simulink model "step_response_firstorder_rl_rc"  (R2021a)
settings: Solver=VariableStepAuto  StartTime=0.0  StopTime=0.05  RelTol=1e-3
libraries: spsSeriesRLCBranchLib x12, spsControlledVoltageSourceLib x6, spsCurrentMeasurementLib x6, spsVoltageMeasurementLib x6, spspowerguiLib x1
settings Model: Creator=LENOVO  LastModifiedBy=LENOVO

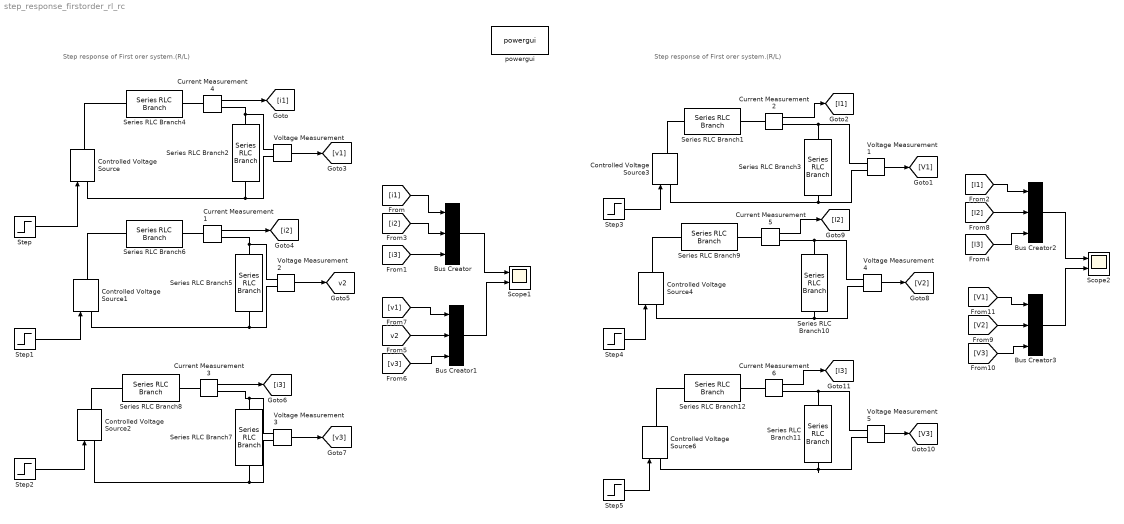
== system step_response_firstorder_rl_rc ==
  note: Step response of First orer system.(R/L)
  note: Step response of First orer system.(R/L)
  Bus Creator{,1..3} (4 alike) : BusCreator  Inputs=3
  Controlled Voltage Source{,1..4,6} (6 alike) : spsControlledVoltageSourceLib/Controlled Voltage Source  Initialize=on  Source_Type=AC  Amplitude=0  Phase=0  Frequency=0  Measurements=None
  Current Measurement{1..6} (6 alike) : spsCurrentMeasurementLib/Current Measurement  PhasorSimulation=off  OutputType=Complex  PSBequivalent=0
  Scope1 : Scope  NumInputPorts=2
  Scope2 : Scope  NumInputPorts=2
  Series RLC Branch1 : spsSeriesRLCBranchLib/Series RLC Branch  LConnTagsString=__new0  RConnTagsString=__new0  BranchType=R  Resistance=1  Inductance=1e-3  SetiL0=off  InitialCurrent=0  Capacitance=1e-6  Setx0=off  InitialVoltage=0  Measurements=None
  Series RLC Branch10 : spsSeriesRLCBranchLib/Series RLC Branch  LConnTagsString=__new0  RConnTagsString=__new0  BranchType=C  Resistance=1  Inductance=1e-3  SetiL0=off  InitialCurrent=0  Capacitance=100e-5  Setx0=off  InitialVoltage=0  Measurements=None
  Series RLC Branch11 : spsSeriesRLCBranchLib/Series RLC Branch  LConnTagsString=__new0  RConnTagsString=__new0  BranchType=C  Resistance=1  Inductance=1e-3  SetiL0=off  InitialCurrent=0  Capacitance=100e-5  Setx0=off  InitialVoltage=0  Measurements=None
  Series RLC Branch12 : spsSeriesRLCBranchLib/Series RLC Branch  LConnTagsString=__new0  RConnTagsString=__new0  BranchType=R  Resistance=5  Inductance=1e-3  SetiL0=off  InitialCurrent=0  Capacitance=1e-6  Setx0=off  InitialVoltage=0  Measurements=None
  Series RLC Branch2 : spsSeriesRLCBranchLib/Series RLC Branch  LConnTagsString=__new0  RConnTagsString=__new0  BranchType=L  Resistance=1  Inductance=5e-3  SetiL0=off  InitialCurrent=0  Capacitance=1e-6  Setx0=off  InitialVoltage=0  Measurements=None
  Series RLC Branch3 : spsSeriesRLCBranchLib/Series RLC Branch  LConnTagsString=__new0  RConnTagsString=__new0  BranchType=C  Resistance=1  Inductance=1e-3  SetiL0=off  InitialCurrent=0  Capacitance=100e-5  Setx0=off  InitialVoltage=0  Measurements=None
  Series RLC Branch4 : spsSeriesRLCBranchLib/Series RLC Branch  LConnTagsString=__new0  RConnTagsString=__new0  BranchType=R  Resistance=1  Inductance=1e-3  SetiL0=off  InitialCurrent=0  Capacitance=1e-6  Setx0=off  InitialVoltage=0  Measurements=None
  Series RLC Branch5 : spsSeriesRLCBranchLib/Series RLC Branch  LConnTagsString=__new0  RConnTagsString=__new0  BranchType=L  Resistance=1  Inductance=5e-3  SetiL0=off  InitialCurrent=0  Capacitance=1e-6  Setx0=off  InitialVoltage=0  Measurements=None
  Series RLC Branch6 : spsSeriesRLCBranchLib/Series RLC Branch  LConnTagsString=__new0  RConnTagsString=__new0  BranchType=R  Resistance=3  Inductance=1e-3  SetiL0=off  InitialCurrent=0  Capacitance=1e-6  Setx0=off  InitialVoltage=0  Measurements=None
  Series RLC Branch7 : spsSeriesRLCBranchLib/Series RLC Branch  LConnTagsString=__new0  RConnTagsString=__new0  BranchType=L  Resistance=1  Inductance=5e-3  SetiL0=off  InitialCurrent=0  Capacitance=1e-6  Setx0=off  InitialVoltage=0  Measurements=None
  Series RLC Branch8 : spsSeriesRLCBranchLib/Series RLC Branch  LConnTagsString=__new0  RConnTagsString=__new0  BranchType=R  Resistance=5  Inductance=1e-3  SetiL0=off  InitialCurrent=0  Capacitance=1e-6  Setx0=off  InitialVoltage=0  Measurements=None
  Series RLC Branch9 : spsSeriesRLCBranchLib/Series RLC Branch  LConnTagsString=__new0  RConnTagsString=__new0  BranchType=R  Resistance=3  Inductance=1e-3  SetiL0=off  InitialCurrent=0  Capacitance=1e-6  Setx0=off  InitialVoltage=0  Measurements=None
  Step{,1..5} (6 alike) : Step  Time=0  SampleTime=0
  Voltage Measurement{,1..5} (6 alike) : spsVoltageMeasurementLib/Voltage Measurement  PhasorSimulation=off  OutputType=Complex  PSBequivalent=0
  powergui : spspowerguiLib/powergui  Priority=1  SimulationMode=Continuous  SampleTime=50e-6  frequency=60  Iterations=50  frequencyindice=0  Pbase=100e6  ErrMax=1e-4  UnitsV=kV  UnitsW=MW  buscounter=0  FunctionMessages=off  echomessages=off  EnableUseOfTLC=off  CurrentSourceSwitches=off  DisableSnubberDevices=off  DisableRonSwitches=off  DisableVfSwitches=off  DisplayEquations=off  AutomaticDiscreteSolvers=off  SolverType=Tustin/Backward Euler (TBE)  Interpol=off  ExternalGateDelay=off  methode=off  Ts=100  x0status=blocks  SPID=on  SwTol=0  HookPort=off  NonlinearTolerance=1e-4  nMaxIteration=100  ContinueOnMaxIteration=off  RestoreLinks=warning  ResistiveCurrentMeasurement=off  Frange=[0:2:500]  Ylog=off  Xlog=on  ShowGrid=off  save=off  variable=ZData  structure=0  ZoomFFT=off  StartTime=0.0  cycles=1  DisplayStyle=1  fundamental=60  FreqAxis=off  MaxFrequency=1000  frequencyindicesteady=1  RmsSteady=1  display=off
  tag scope: v2=global
  wires:
  Voltage Measurement/1 -> [v1]
  Current Measurement4/1 -> [i1]
  Current Measurement2/1 -> [I1]
  Voltage Measurement1/1 -> [V1]
  Current Measurement1/1 -> [i2]
  Voltage Measurement3/1 -> [v3]
  Current Measurement3/1 -> [i3]
  Voltage Measurement4/1 -> [V2]
  Current Measurement5/1 -> [I2]
  Current Measurement6/1 -> [I3]
  Voltage Measurement5/1 -> [V3]
  Bus Creator2/1 -> Scope2/1
  Bus Creator3/1 -> Scope2/2
  Bus Creator/1 -> Scope1/1
  Bus Creator1/1 -> Scope1/2
  [i1] -> Bus Creator/1
  [i2] -> Bus Creator/2
  [i3] -> Bus Creator/3
  [v1] -> Bus Creator1/1
  [v3] -> Bus Creator1/3
  [I1] -> Bus Creator2/1
  [I2] -> Bus Creator2/2
  [I3] -> Bus Creator2/3
  [V1] -> Bus Creator3/1
  [V2] -> Bus Creator3/2
  [V3] -> Bus Creator3/3
  Voltage Measurement2/1 -> [v2]
  [v2] -> Bus Creator1/2
  Step/1 -> Controlled Voltage Source/1
  Step5/1 -> Controlled Voltage Source6/1
  Step4/1 -> Controlled Voltage Source4/1
  Step3/1 -> Controlled Voltage Source3/1
  Step1/1 -> Controlled Voltage Source1/1
  Step2/1 -> Controlled Voltage Source2/1
  connections:
  Controlled Voltage Source/RConn1 -- Series RLC Branch4/LConn1
  Current Measurement4/LConn1 -- Series RLC Branch4/RConn1
  Series RLC Branch2/LConn1 -- Voltage Measurement/LConn1 -- Current Measurement4/RConn1
  Series RLC Branch2/RConn1 -- Controlled Voltage Source/LConn1 -- Voltage Measurement/LConn2
  Controlled Voltage Source3/RConn1 -- Series RLC Branch1/LConn1
  Voltage Measurement1/LConn2 -- Controlled Voltage Source3/LConn1 -- Series RLC Branch3/RConn1
  Current Measurement2/LConn1 -- Series RLC Branch1/RConn1
  Current Measurement2/RConn1 -- Series RLC Branch3/LConn1 -- Voltage Measurement1/LConn1
  Voltage Measurement2/LConn1 -- Series RLC Branch5/LConn1 -- Current Measurement1/RConn1
  Voltage Measurement2/LConn2 -- Controlled Voltage Source1/LConn1 -- Series RLC Branch5/RConn1
  Series RLC Branch6/LConn1 -- Controlled Voltage Source1/RConn1
  Current Measurement1/LConn1 -- Series RLC Branch6/RConn1
  Series RLC Branch7/LConn1 -- Current Measurement3/RConn1 -- Voltage Measurement3/LConn1
  Series RLC Branch7/RConn1 -- Controlled Voltage Source2/LConn1 -- Voltage Measurement3/LConn2
  Current Measurement3/LConn1 -- Series RLC Branch8/RConn1
  Series RLC Branch8/LConn1 -- Controlled Voltage Source2/RConn1
  Voltage Measurement4/LConn2 -- Controlled Voltage Source4/LConn1 -- Series RLC Branch10/RConn1
  Series RLC Branch10/LConn1 -- Voltage Measurement4/LConn1 -- Current Measurement5/RConn1
  Current Measurement5/LConn1 -- Series RLC Branch9/RConn1
  Controlled Voltage Source4/RConn1 -- Series RLC Branch9/LConn1
  Series RLC Branch11/RConn1 -- Controlled Voltage Source6/LConn1 -- Voltage Measurement5/LConn2
  Voltage Measurement5/LConn1 -- Series RLC Branch11/LConn1 -- Current Measurement6/RConn1
  Current Measurement6/LConn1 -- Series RLC Branch12/RConn1
  Controlled Voltage Source6/RConn1 -- Series RLC Branch12/LConn1
